simulink model "untitled1"  (R2024b)
settings: Solver=VariableStepAuto  StartTime=0.0  StopTime=10.0  RelTol=1e-3
settings Model: Creator=sushm  LastModifiedBy=sushm

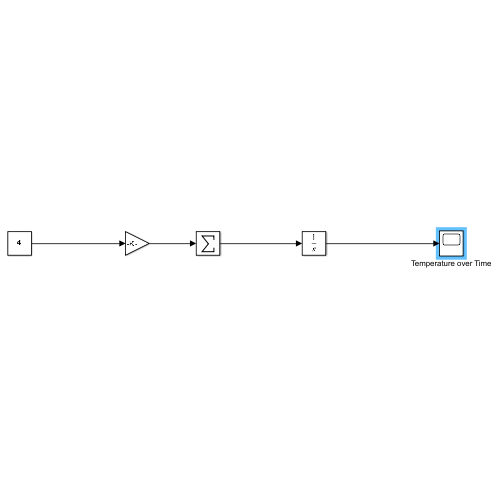
[thumbnail: Simulink's stored preview of the top-level diagram]
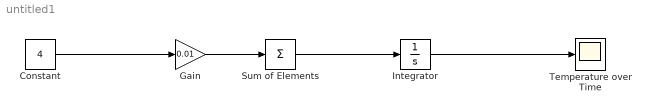
== system untitled1 ==
  Constant : Constant  Value=4
  Gain : Gain  Gain=0.01
  Integrator : Integrator  InitialCondition=1
  Sum of Elements : Sum  Inputs=+
  Temperature over Time : Scope
  wires:
  Constant/1 -> Gain/1
  Integrator/1 -> Temperature over Time/1
  Sum of Elements/1 -> Integrator/1
  Gain/1 -> Sum of Elements/1
